simulink model "Suspension"  (R2020b)
settings: Solver=VariableStepAuto  StartTime=0.0  StopTime=10.0  RelTol=1e-3
settings Model: Creator=Akshata Ashok  LastModifiedBy=Akshata Ashok

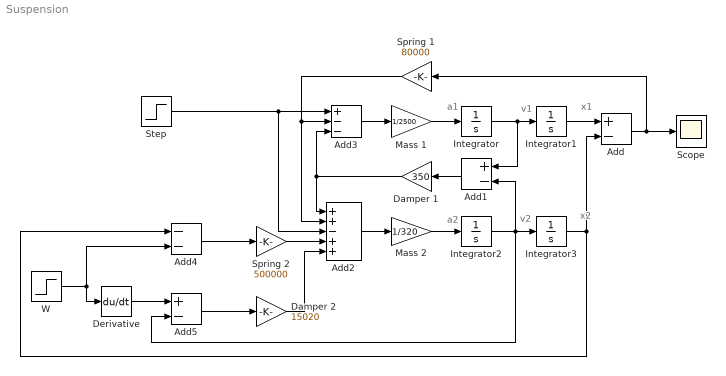
== system Suspension ==
  note: v1
  note: v2
  note: a2
  note: x1
  note: x2
  note: a1
  Add : Sum  Inputs=+-
  Add1 : Sum  Inputs=+-
  Add2 : Sum  Inputs=++-++
  Add3 : Sum  Inputs=+--
  Add4 : Sum  Inputs=--
  Add5 : Sum  Inputs=+-
  Damper 1 : Gain  Gain=350
  Damper 2 : Gain  Gain=15020
  Derivative : Derivative
  Integrator{,1..3} (4 alike) : Integrator
  Mass 1 : Gain  Gain=1/2500
  Mass 2 : Gain  Gain=1/320
  Scope : Scope
  Spring 1 : Gain  Gain=80000
  Spring 2 : Gain  Gain=500000
  Step : Step  Time=0  SampleTime=0
  W : Step  Time=0  After=0
  wires:
  Integrator3/1 -> Add/2, Add4/1
  Add4/1 -> Spring 2/1
  Integrator/1 -> Add1/1, Integrator1/1
  Mass 1/1 -> Integrator/1
  Integrator2/1 -> Add5/2, Add1/2, Integrator3/1
  Add/1 -> Scope/1, Spring 1/1
  Mass 2/1 -> Integrator2/1
  Integrator1/1 -> Add/1
  Add1/1 -> Damper 1/1
  Add2/1 -> Mass 2/1
  Add3/1 -> Mass 1/1
  Damper 1/1 -> Add3/3, Add2/1
  Spring 1/1 -> Add3/2, Add2/2
  Damper 2/1 -> Add2/5
  Spring 2/1 -> Add2/4
  Derivative/1 -> Add5/1
  Add5/1 -> Damper 2/1
  W/1 -> Add4/2, Derivative/1
  Step/1 -> Add3/1, Add2/3
